simulink library "vrlib"  (Simulink 6.0)
settings: Solver=ode45  SolverMode=SingleTasking  StartTime=0.0  StopTime=10.0  RelTol=1e-3
undefined symbols (not defined in the file or in its folder): gcbh, vrmfunc
libraries: vrlib x1
settings Model: CovMetricSettings=d  Creator=Dluhos  LastModifiedBy=Houska
settings DataIOCC: SignalLoggingName=logsOut
settings OptimizationCC: BooleanDataType=off
settings DebuggingCC: CheckExecutionContextPreStartOutputMsg=on  CheckExecutionContextRuntimeOutputMsg=on  SolverPrmCheckMsg=none
settings HardwareCC: TargetUnknown=on
settings ModelReferenceCC: UpdateModelReferenceTargets=IfOutOfDate
settings GRTTargetCC: LifeSpan=inf
settings SFSimCC: SFSimApplyToAllLibs=on  SFSimBuildMode=Incremental

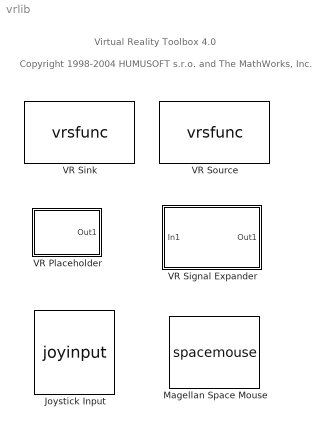
== system vrlib ==
  note: Copyright 1998-2004 HUMUSOFT s.r.o. and The MathWorks, Inc.
  note: Virtual Reality Toolbox 4.0
  Joystick Input : S-Function  FunctionName=joyinput  Parameters=joyid, adjustports, forcefeed  mask(Joystick Input){joyid=1, adjustports=on, forcefeed=off}
      mask prompts: joyid "Joystick ID:"; adjustports "Adjust I/O ports according to joystick capabilities"; forcefeed "Enable force-feedback input"
      mask help: Joystick input device driver.
      mask Help: helpview(fullfile(docroot, 'toolbox', 'vr', 'vr.map'), 'vr_joystickinput');
      mask Display:
      | image(imread('joystickicon.png'));
      | port_label('output', 1, 'Axes');
      | port_label('output', 2, 'Buttons');
      | port_label('output', 3, 'Point of View');
  Magellan Space Mouse : S-Function  FunctionName=spacemouse  Parameters=Port, OutputType, InitialPosition, InitialRotation, PositionSensitivity, RotationSensitivity, Dominant, NormalizeAngle, DisableTranslation, DisableRotation  mask(Magellan Space Mouse){Port=COM1, OutputType=Speed, Dominant=off, DisableTranslation=off, DisableRotation=off, NormalizeAngle=off, PositionSensitivity=0.0001, RotationSensitivity=0.00001, InitialPosition=[0 0 0], InitialRotation=[0 0 1 0]}
      mask prompts: OutputType "Output type:"; Dominant "Dominant mode"; DisableTranslation "Disable position movement"; DisableRotation "Disable rotation movement"; NormalizeAngle "Normalize output angle"; PositionSensitivity "Position sensitivity:"; RotationSensitivity "Rotation sensitivity:"; InitialPosition "Initial position:"; InitialRotation "Initial rotation:"
      mask help: Magellan Space Mouse input device driver.
      mask Help: helpview(fullfile(docroot, 'toolbox', 'vr', 'vr.map'), 'vr_magellanspacemouse');
      mask StyleString: popup(COM1|COM2|COM3|COM4|USB),popup(Speed|Position|Viewpoint coordinates),checkbox,checkbox,checkbox,checkbox,edit,edit,edit,edit
      mask CallbackString: |spacemousemask||||||||
      mask Display:
      | image(imread('spacemouseicon.png'))
      | port_label('output', 1, 'Translation')
      | port_label('output', 2, 'Rotation')
      | port_label('output', 3, 'Buttons')
  VR Placeholder : Subsystem  EnableExecutionContextPropagation=on  mask(VR Placeholder){outwidth=1}
      mask prompts: outwidth "Output width"
      mask help: Generate a vector of VR Placeholder signals used for masking the unused or unaffected components of VRML fields.
      mask Help: helpview(fullfile(docroot, 'toolbox', 'vr', 'vr.map'), 'vr_vrplaceholder');
      mask Display:
      | text(0.1,0.5,'VR');
      | plot([0.4 0.4], [0.3 0.7]);
      | plot([0.4 0.9], [0.45 0.44]);
      | plot([0.4 0.9], [0.5 0.5]);
      | plot([0.4 0.9], [0.55 0.55]);
  VR Signal Expander : Subsystem  EnableExecutionContextPropagation=on  mask(VR Signal Expander){outwidth=4, outidx=[2 4]}
      mask prompts: outwidth "Output width"; outidx "Output signal indices"
      mask help:
      | Expand input vector into a fully qualified VRML field signal, filling the blank positions in the output port with the VR Placeholder signal.
      |
      | Input: The vector of inputs to be mapped into the output port.
      | Output width: The width of the output port.
      | Output signal indices: Positions of output vector at which the input signal elements appear. The remaining positions are filled with the VR Placeholder signal.
      mask init:
      | sel=ones(1,outwidth);
      | sel(outidx)=2:(length(outidx)+1);
      mask Help: helpview(fullfile(docroot, 'toolbox', 'vr', 'vr.map'), 'vr_vrsignalexpander');
      mask Display:
      | text(0.13,0.2,'VR');
      | plot([0.1 0.9],[0.6 0.9]);
      | plot([0.1 0.9],[0.55 0.8]);
      | plot([0.1 0.9],[0.5 0.5]);
      | plot([0.1 0.9],[0.45 0.2]);
      | plot([0.1 0.9],[0.4 0.1]);
  VR Sink : S-Function  LoadFcn=vrmfunc('FnLoad', gcbh);  InitFcn=vrmfunc('FnInit', gcbh);  FunctionName=vrsfunc  Parameters=WorldFileName, {}, FieldsWritten, AutoView, RemoteView, RemoteChange, SampleTime, WorldDescription  mask(Virtual Reality Sink){SampleTime=0.1, ViewEnable=on, RemoteChange=off, RemoteView=on, FieldsWritten=, WorldFileName=, WorldDescription=, AutoView=off, FigureProperties={}}
      mask prompts: SampleTime "Sample Time"; ViewEnable "View"; RemoteChange "Remote Change"; RemoteView "Remote View"; FieldsWritten "Fields Written"; WorldFileName "World File Name"; WorldDescription "World Description"; FigureProperties "Figure Properties"
      mask help: Controls the selected fields of a virtual world according to given inputs.
      mask init:
      | set_param(gcbh, 'MaskDisplay', vrmfunc('FnIcon'));
      settings: CopyFcn=vrmfunc('FnCopy', gcbh);  DeleteFcn=vrmfunc('FnDelete', gcbh);  PreSaveFcn=vrmfunc('FnPreSave', gcbh);  DestroyFcn=vrmfunc('FnDestroy', gcbh);  OpenFcn=vrmfunc('FnOpen', gcbh);  CloseFcn=vrmfunc('FnClose', gcbh);
      mask Help: helpview(fullfile(docroot, 'toolbox', 'vr', 'vr.map'), 'vr_vrsink');
      mask Display: image(imread('vrblockicon.png'))
  VR Source : S-Function  LoadFcn=vrmfunc('FnLoad', gcbh);  InitFcn=vrmfunc('FnInit', gcbh);  FunctionName=vrsfunc  Parameters=WorldFileName, FieldsRead, {}, AutoView, RemoteView, RemoteChange, SampleTime, WorldDescription  mask(Virtual Reality Source){SampleTime=0.1, ViewEnable=on, RemoteChange=off, RemoteView=on, FieldsRead=, WorldFileName=, WorldDescription=, AutoView=off, FigureProperties={}}
      mask prompts: SampleTime "Sample Time"; ViewEnable "View"; RemoteChange "Remote Change"; RemoteView "Remote View"; FieldsRead "Fields Written"; WorldFileName "World File Name"; WorldDescription "World Description"; FigureProperties "Figure Properties"
      mask help: Reads the selected fields of a virtual world.
      mask init:
      | set_param(gcbh, 'MaskDisplay', vrmfunc('FnIcon'));
      settings: CopyFcn=vrmfunc('FnCopy', gcbh);  DeleteFcn=vrmfunc('FnDelete', gcbh);  PreSaveFcn=vrmfunc('FnPreSave', gcbh);  DestroyFcn=vrmfunc('FnDestroy', gcbh);  OpenFcn=vrmfunc('FnOpen', gcbh);  CloseFcn=vrmfunc('FnClose', gcbh);
      mask Help: helpview(fullfile(docroot, 'toolbox', 'vr', 'vr.map'), 'vr_vrsource');
      mask Display: image(imread('vrblockicon.png'))

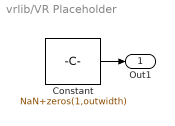
== system vrlib/VR Placeholder ==
  Constant : Constant  Value=NaN+zeros(1,outwidth)
  Out1 : Outport
  wires:
  Constant/1 -> Out1/1

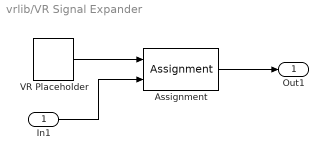
== system vrlib/VR Signal Expander ==
  In1 : Inport  LatchInput=off
  Assignment : Assignment  Elements=outidx
  VR Placeholder : vrlib/VR Placeholder  outwidth=outwidth
  Out1 : Outport
  wires:
  Assignment/1 -> Out1/1
  VR Placeholder/1 -> Assignment/1
  In1/1 -> Assignment/2
